simulink model "PolePlaceHeliIntegerObsv"  (R2021a)
settings: Solver=VariableStepAuto  StartTime=0.0  StopTime=10.0  MaxStep=1e-3  RelTol=1e-3
values from neighbouring files (symbols this model uses):
  A = [0 0 1 0 ... (first row only)    [HeliControlGain.m]    (also in HeliControlHinf.m; HeliControlInteger.m; HeliControlLQG.m; HeliControlLQRgain.m)
  Aoss = A-L*C    [HeliControlIntegerObsv.m]
  B = [0 0 ... (first row only)    [HeliControlGain.m]    (also in HeliControlHinf.m; HeliControlInteger.m; HeliControlLQG.m; HeliControlLQRgain.m)
  Boss = [B-L*D L]    [HeliControlIntegerObsv.m]
  C = [1 0 0 0 ... (first row only)    [HeliControlGain.m]    (also in HeliControlHinf.m; HeliControlInteger.m; HeliControlLQG.m; HeliControlLQRgain.m)
  Coss = eye(4)    [HeliControlIntegerObsv.m]
  D = zeros(2,2)    [HeliControlGain.m]    (also in HeliControlHinf.m; HeliControlInteger.m; HeliControlLQG.m; HeliControlLQRgain.m)
  Doss = zeros(4,4)    [HeliControlIntegerObsv.m]
  Kf = K(:,1:4)    [HeliControlInteger.m]    (also in HeliControlIntegerObsv.m; HeliControlLQG.m; HeliControlLQRinteger.m)
  Ki = K(:,5:end)    [HeliControlInteger.m]    (also in HeliControlIntegerObsv.m; HeliControlLQG.m; HeliControlLQRinteger.m)
settings Model: Creator=Ciro  LastModifiedBy=Ciro

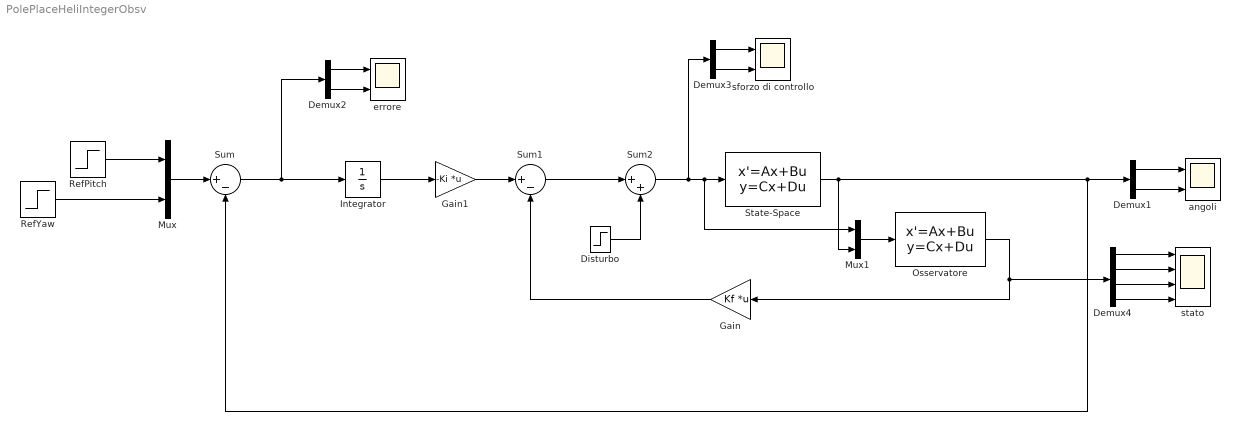
== system PolePlaceHeliIntegerObsv ==
  Demux1 : Demux  Outputs=2
  Demux2 : Demux  Outputs=2
  Demux3 : Demux  Outputs=2
  Demux4 : Demux
  Disturbo : Step  Time=6  SampleTime=0
  Gain : Gain  Gain=Kf  Multiplication=Matrix(K*u)
  Gain1 : Gain  Gain=-Ki  Multiplication=Matrix(K*u)
  Integrator : Integrator
  Mux : Mux  Inputs=2
  Mux1 : Mux  Inputs=2
  Osservatore : StateSpace  A=Aoss  B=Boss  C=Coss  D=Doss  InitialCondition=[0.1;0.1;0;0]  ParameterTunability=Optimized
  RefPitch : Step  Time=0.1  After=0.3  SampleTime=0
  RefYaw : Step  Time=0.1  After=0.3  SampleTime=0
  State-Space : StateSpace  A=A  B=B  C=C  D=D  InitialCondition=0
  Sum : Sum  Inputs=|+-
  Sum1 : Sum  Inputs=|+-
  Sum2 : Sum  Inputs=|++
  angoli : Scope  NumInputPorts=2
  errore : Scope  NumInputPorts=2
  sforzo di controllo : Scope  NumInputPorts=2
  stato : Scope  NumInputPorts=4
  wires:
  Integrator/1 -> Gain1/1
  RefPitch/1 -> Mux/1
  RefYaw/1 -> Mux/2
  Mux/1 -> Sum/1
  Sum/1 -> Demux2/1, Integrator/1
  Gain1/1 -> Sum1/1
  Gain/1 -> Sum1/2
  Sum1/1 -> Sum2/1
  Sum2/1 -> Demux3/1, Mux1/1, State-Space/1
  Disturbo/1 -> Sum2/2
  State-Space/1 -> Mux1/2, Demux1/1, Sum/2
  Demux1/1 -> angoli/1
  Demux1/2 -> angoli/2
  Demux2/1 -> errore/1
  Demux2/2 -> errore/2
  Demux3/1 -> sforzo di controllo/1
  Demux3/2 -> sforzo di controllo/2
  Mux1/1 -> Osservatore/1
  Demux4/1 -> stato/1
  Osservatore/1 -> Gain/1, Demux4/1
  Demux4/2 -> stato/2
  Demux4/3 -> stato/3
  Demux4/4 -> stato/4
